simulink model "ssc_opamp_bandlimited"  (R2020b)
settings: Solver=VariableStepAuto  StartTime=0.0  StopTime=0.02  MaxStep=0.0001  RelTol=1e-3  AbsTol=1e-3  EnableMultiTasking=on
libraries: fl_lib x14, nesl_utility x3
CloseFcn:
  | try,close(h1_ssc_opamp_bandlimited),end
  | clear h1_ssc_opamp_bandlimited
  | clear simlog_ssc_opamp_bandlimited
Description:
  | Band-Limited Op-Amp
  | 
  | Copyright 2008-2018 The MathWorks, Inc.
settings Model: Creator=MathWorks  LastModifiedBy=bolic
settings SolverCC: AutoScaleAbsTol=off
settings DataIOCC: LimitDataPoints=on  SaveFormat=Array  ReturnWorkspaceOutputs=off
settings OptimizationCC: LifeSpan=inf
settings DebuggingCC: SolverPrmCheckMsg=warning  AllowSymbolicDim=off  SFUnexpectedBacktrackingDiag=warning  SFNoUnconditionalDefaultTransitionDiag=warning  SFExecutionAtInitializationDiag=none  ArithmeticOperatorsInVariantConditions=warning
settings HardwareCC: ProdBitPerPointer=32  ProdBitPerSizeT=32  ProdBitPerPtrDiffT=32  ProdLargestAtomicFloat=None  ProdIntDivRoundTo=Undefined  ProdEndianess=Unspecified  ProdWordSize=32  ProdHWDeviceType=32-bit Generic
settings ModelReferenceCC: PropagateSignalLabelsOutOfModel=off
settings SFSimCC: SimUseLocalCustomCode=off  CustomCodeUndefinedFunction=UseInterfaceOnly
settings RTWCC: RTWUseLocalCustomCode=off
settings CodeAppCC: StateflowObjectComments=on
settings GRTTargetCC: TargetLangStandard=C89/C90 (ANSI)
settings ConfigComp: CovMetricSettings=dw  CovSaveCumulativeToWorkspaceVar=on  CovSaveSingleToWorkspaceVar=on  CovExternalEMLEnable=off  CovSFcnEnable=off
settings SimscapeCC: SimscapeLogType=all  SimscapeLogSimulationStatistics=on  SimscapeLogName=simlog_ssc_opamp_bandlimited  SimscapeLogDataHistory=10000

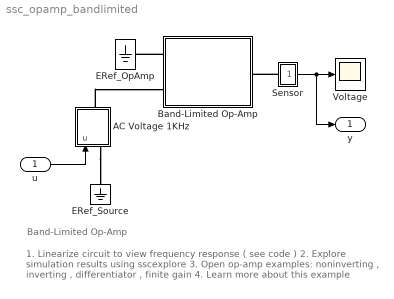
== system ssc_opamp_bandlimited ==
  note: 1. Linearize circuit to view frequency response ( see code )
      | 2. Explore simulation results using sscexplore
      | 3. Open op-amp examples:
      | noninverting , inverting , differentiator , finite gain
      | 4. Learn more about this example
  note: Band-Limited Op-Amp
  u : Inport
  AC Voltage 1KHz : Subsystem
  Band-Limited Op-Amp : Subsystem  Tag=PublishSubsystem
      mask Display:
      | % Plot Op-Amp
      | plot([1,2,1,1],[1,2,3,1])
      | %color('red')
      | %plot([1.5 1.5],[1.5 1.1])
      | %plot([1.35 1.65],[1.1 1.1])
      | %plot([1.4 1.6],[1 1])
      | %plot([1.45 1.55],[0.9 0.9])
      | %color('black')
      | 
      | % Band-limited symbol
      | % 'B'
      | plot([1.1,1.1],[1.7,2.2])
      | plot([1.1,1.2,1.25,1.27,1.27,1.25,1.2,1.1],[2.2,2.2,2.15,2.1,2.1,2.0,1.95,1.95])
      | plot([1.1,1.2,1.25,1.27,1.27,1.25,1.2,1.1],[2.2,2.2,2.15,2.1,2.1,2.0,1.95,1.95]-0.25)
      | 
      | % 'W'
      | plot([1.35,1.35,1.5],[2.2,1.7,1.7])
      | 
      | 
      | %  Connection
      | plot([2,2.5],[2,2])
      | plot([0.5, 1],[1.45 1.45])
      | plot([0.5, 1],[2.75 2.75])
      | 
      | % Scaling
      | color('white')
      | plot(0.5,0.8)
      | plot(2.5,3.4)
      | 
      | color('red')
      | port_label('LConn',1,'+');
      | port_label('LConn',2,'-');
  ERef_OpAmp : fl_lib/Electrical/Electrical Elements/Electrical Reference
  ERef_Source : fl_lib/Electrical/Electrical Elements/Electrical Reference
  Sensor : Subsystem
      mask Display: disp('S')
  Voltage : Scope
  y : Outport  VectorParamsAs1DForOutWhenUnconnected=off
  wires:
  Sensor/1(Out1) -> Voltage/1, y/1
  u/1 -> AC Voltage 1KHz/1(u)
  connections:
  AC Voltage 1KHz/LConn1 -- ERef_Source/LConn1
  Band-Limited Op-Amp/LConn1 -- ERef_OpAmp/LConn1
  Sensor/LConn1 -- Band-Limited Op-Amp/RConn1
  AC Voltage 1KHz/RConn1 -- Band-Limited Op-Amp/LConn2

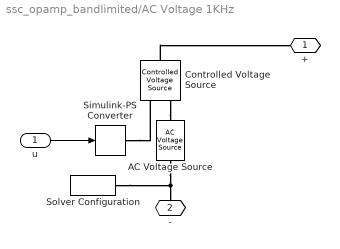
== system ssc_opamp_bandlimited/AC Voltage 1KHz ==
  u : Inport
  AC Voltage Source : fl_lib/Electrical/Electrical Sources/AC Voltage Source  amp=1e-5 V  shift=0 deg  frequency=1000 Hz  omega=0 rad/s
  Controlled Voltage Source : fl_lib/Electrical/Electrical Sources/Controlled Voltage Source
  Simulink-PS Converter : nesl_utility/Simulink-PS Converter  PhysicalDomain=network_engine_domain  SubClassName=ps_input  LeftPortType=input  RightPortType=output  PseudoPeriodic=off  Frequencies=[]  NoiseDistribution=none  NoiseParameters=[]  Unit=V  AffineConversion=off  FilteringAndDerivatives=zero  SimscapeFilterOrder=1  InputFilterTimeConstant=.001  UdotUserProvided=0
  Solver Configuration : nesl_utility/Solver Configuration  PhysicalDomain=network_engine_domain  SubClassName=solver  LeftPortType=input  RightPortType=generic  Tones=[]  Harmonics=[]  SimulateNoise=off  Profile=off  UseLocalSampling=off  EnableSwitchedLinearOptims=on  FrequencyDomain=off  UseCCode=off  RelTol=0.001  AbsTol=1e-06  MinStep=1e-09  ToWorkspace=off  RevertToSquareIcSolve=off  NumHomotopyIterations=100  PhasorMode=off  PhasorModeNumHarmonics=1  DoDC=on  ResidualTolerance=1e-9  UseLocalSolver=off  LocalSolverChoice=NE_BACKWARD_EULER_ADVANCER  LocalSolverSampleTime=.001  DoFixedCost=off  MaxNonlinIter=3  MaxModeIter=2  ComputeImpulses=off  ImpulseIterations=2  LinearAlgebra=auto  EquationFormulation=NE_TIME_EF  DelaysMemoryBudget=1024  AutomaticFiltering=on  FilteringTimeConstant=0.001  PartitionStorageMethod=AS_NEEDED  PartitionMemoryBudget=1024  PartitionMethod=FAST
  + : PMIOPort  Side=Right
  - : PMIOPort  Port=2  Side=Left
  wires:
  u/1 -> Simulink-PS Converter/1
  connections:
  AC Voltage Source/RConn1 -- Solver Configuration/RConn1 -- -/RConn1
  Controlled Voltage Source/RConn2 -- AC Voltage Source/LConn1
  Simulink-PS Converter/RConn1 -- Controlled Voltage Source/RConn1
  Controlled Voltage Source/LConn1 -- +/RConn1

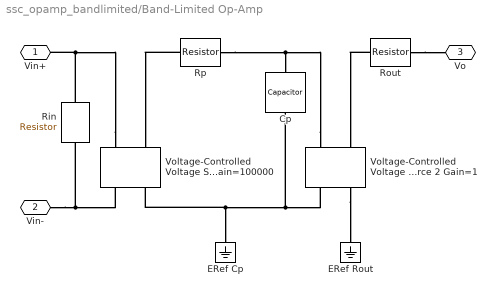
== system ssc_opamp_bandlimited/Band-Limited Op-Amp ==
  Cp : fl_lib/Electrical/Electrical Elements/Capacitor  Tag=Factory Generic  c=1.5915 nF  r=1e-06 Ohm  g=0 1/Ohm  i_specify=off  i_priority=High  i=0 A  i_nominal_specify=off  i_nominal_unit=A  i_nominal_value=1  v_specify=off  v_priority=High  v=0 V  v_nominal_specify=off  v_nominal_unit=V  v_nominal_value=1  vc_specify=on  vc_priority=High  vc=0 V  vc_nominal_specify=off  vc_nominal_unit=V  vc_nominal_value=1
      settings: AttributesFormatString=|
      | %<c>
      | %<c_unit>
  ERef Cp : fl_lib/Electrical/Electrical Elements/Electrical Reference  Tag=Factory Generic
  ERef Rout : fl_lib/Electrical/Electrical Elements/Electrical Reference  Tag=Factory Generic
  Rin : fl_lib/Electrical/Electrical Elements/Resistor  Tag=Factory Generic  R=100 kOhm  i_specify=off  i_priority=High  i=0 A  i_nominal_specify=off  i_nominal_unit=A  i_nominal_value=1  v_specify=off  v_priority=High  v=0 V  v_nominal_specify=off  v_nominal_unit=V  v_nominal_value=1
      settings: AttributesFormatString=|
      | %<R>
      | %<R_unit>
  Rout : fl_lib/Electrical/Electrical Elements/Resistor  Tag=Factory Generic  R=10 Ohm  i_specify=off  i_priority=High  i=0 A  i_nominal_specify=off  i_nominal_unit=A  i_nominal_value=1  v_specify=off  v_priority=High  v=0 V  v_nominal_specify=off  v_nominal_unit=V  v_nominal_value=1
      settings: AttributesFormatString=|
      | %<R>
      | %<R_unit>
  Rp : fl_lib/Electrical/Electrical Elements/Resistor  Tag=Factory Generic  R=100 kOhm  i_specify=off  i_priority=High  i=0 A  i_nominal_specify=off  i_nominal_unit=A  i_nominal_value=1  v_specify=off  v_priority=High  v=0 V  v_nominal_specify=off  v_nominal_unit=V  v_nominal_value=1
      settings: AttributesFormatString=|
      | %<R>
      | %<R_unit>
  Voltage-Controlled Voltage Source 1 Gain=100000 : fl_lib/Electrical/Electrical Sources/Voltage-Controlled Voltage Source  K=100000  v1_specify=off  v1_priority=High  v1=0 V  v1_nominal_specify=off  v1_nominal_unit=V  v1_nominal_value=1  v2_specify=off  v2_priority=High  v2=0 V  v2_nominal_specify=off  v2_nominal_unit=V  v2_nominal_value=1
      settings: SourceProductBaseCode=SS  InternalSimscapePortConfiguration="{\"Bottom\":[],\"Left\":[{\"id\":\"p1\",\"label\":\"+\",\"type\":\"foundation.electrical.electrical\"},{\"id\":\"p2\",\"label\":\"+\",\"type\":\"foundation.electrical.electrical\"}],\"Right\":[{\"id\":\"n1\",\"label\":\"-\",\"type\":\"foundation.electrical.electrical\"},{\"id\":\"n2\",\"label\":\"-\",\"type\":\"foundation.electrical.electrical\"}],\"Top\":[]}"
  Voltage-Controlled Voltage Source 2 Gain=1 : fl_lib/Electrical/Electrical Sources/Voltage-Controlled Voltage Source  K=1  v1_specify=off  v1_priority=High  v1=0 V  v1_nominal_specify=off  v1_nominal_unit=V  v1_nominal_value=1  v2_specify=off  v2_priority=High  v2=0 V  v2_nominal_specify=off  v2_nominal_unit=V  v2_nominal_value=1
      settings: SourceProductBaseCode=SS  InternalSimscapePortConfiguration="{\"Bottom\":[],\"Left\":[{\"id\":\"p1\",\"label\":\"+\",\"type\":\"foundation.electrical.electrical\"},{\"id\":\"p2\",\"label\":\"+\",\"type\":\"foundation.electrical.electrical\"}],\"Right\":[{\"id\":\"n1\",\"label\":\"-\",\"type\":\"foundation.electrical.electrical\"},{\"id\":\"n2\",\"label\":\"-\",\"type\":\"foundation.electrical.electrical\"}],\"Top\":[]}"
  Vin+ : PMIOPort  Side=Left
  Vin- : PMIOPort  Port=2  Side=Left
  Vo : PMIOPort  Port=3  Side=Right
  connections:
  Voltage-Controlled Voltage Source 1 Gain=100000/LConn1 -- Rin/LConn1 -- Vin+/RConn1
  Voltage-Controlled Voltage Source 1 Gain=100000/RConn1 -- Vin-/RConn1 -- Rin/RConn1
  Voltage-Controlled Voltage Source 2 Gain=1/LConn1 -- Rp/LConn1 -- Cp/LConn1
  Voltage-Controlled Voltage Source 2 Gain=1/RConn1 -- ERef Cp/LConn1 -- Voltage-Controlled Voltage Source 1 Gain=100000/RConn2 -- Cp/RConn1
  Rout/RConn1 -- Voltage-Controlled Voltage Source 2 Gain=1/LConn2
  Voltage-Controlled Voltage Source 2 Gain=1/RConn2 -- ERef Rout/LConn1
  Rout/LConn1 -- Vo/RConn1
  Rp/RConn1 -- Voltage-Controlled Voltage Source 1 Gain=100000/LConn2

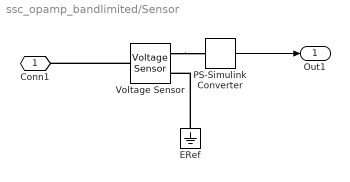
== system ssc_opamp_bandlimited/Sensor ==
  ERef : fl_lib/Electrical/Electrical Elements/Electrical Reference
  PS-Simulink Converter : nesl_utility/PS-Simulink Converter  PhysicalDomain=network_engine_domain  SubClassName=ps_output  LeftPortType=input  RightPortType=output  PseudoPeriodic=off  Frequencies=[]  Unit=1  AffineConversion=off
  Voltage Sensor : fl_lib/Electrical/Electrical Sensors/Voltage Sensor
  Conn1 : PMIOPort  Side=Left
  Out1 : Outport  VectorParamsAs1DForOutWhenUnconnected=off
  wires:
  PS-Simulink Converter/1 -> Out1/1
  connections:
  Voltage Sensor/LConn1 -- Conn1/RConn1
  Voltage Sensor/RConn1 -- PS-Simulink Converter/LConn1
  ERef/LConn1 -- Voltage Sensor/RConn2
